simulink subsystem "moteur_bras_brushless"  (R2024a)
settings: Solver=VariableStepAuto  StartTime=0.0  StopTime=10.0  RelTol=1e-3
undefined symbols (not defined in the file): C_ref, Jv, rpm__max, Vref
libraries: fl_lib x22, fl_ps_legacy_lib x16, nesl_utility x15, sdl_lib x1, ee_lib x1
settings Model: Creator=vincp  LastModifiedBy=VincentPERRET

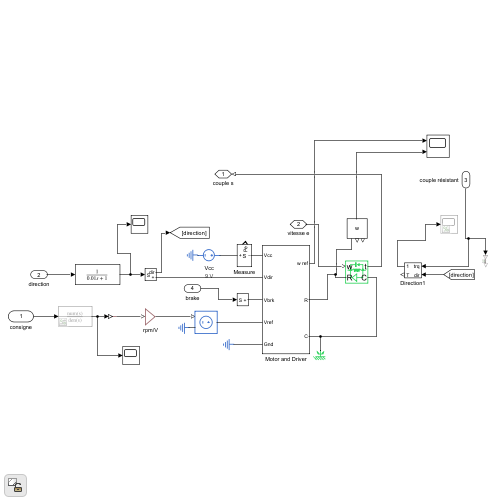
[thumbnail: Simulink's stored preview of the top-level diagram]
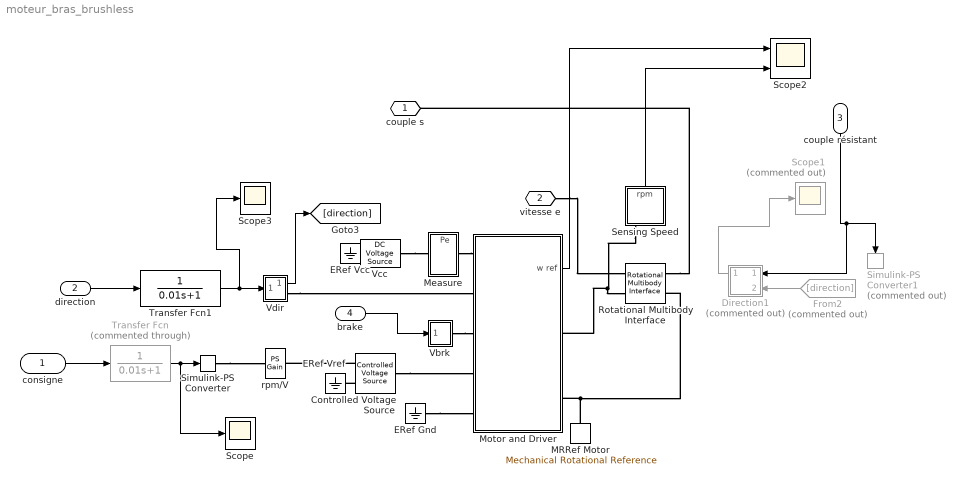
== system moteur_bras_brushless ==
  consigne : Inport
  direction : Inport  Port=2
  couple résistant : Inport  Port=3
  brake : Inport  Port=4
  Controlled Voltage Source : fl_lib/Electrical/Electrical Sources/Controlled Voltage Source
  Direction1 : Subsystem  Commented=on
  ERef Vcc : fl_lib/Electrical/Electrical Elements/Electrical Reference
  ERef Vref : fl_lib/Electrical/Electrical Elements/Electrical Reference
  ERef Gnd : fl_lib/Electrical/Electrical Elements/Electrical Reference
  From2 : From  Commented=on  GotoTag=direction
  MRRef Motor : fl_lib/Mechanical/Rotational Elements/Mechanical Rotational Reference
  Measure : Subsystem
      settings: PortSchema="{\"entries\":[{\"content\":{\"sides\":[{\"content\":{\"connectorIds\":[\"LConn1\"]},\"type\":\"ConnectorPlacement.EquallySpacedRectSide\",\"uuid\":\"8701fb7a-b552-4b0f-ba6a-9ffd5f92813c\"},{\"content\":{\"connectorIds\":[\"RConn1\"],\"side\":\"RIGHT\"},\"type\":\"ConnectorPlacement.EquallySpacedRectSide\",\"uuid\":\"c50126bd-8d71-4912-8eb9-bd6b1a4f4141\"},{\"content\":{\"connectorIds\":[\"Out1\"],\"side\":\"TOP\"},\"type\":\"ConnectorPlacement.EquallySpacedRectSide\",\"uuid\":\"9d2639c5-7e76-4bbd-8c8b-b1e420468010\"}]},\"type\":\"ConnectorPlacement.EquallySpacedConnector\",\"uuid\":\"8f301b36-1aea-45f7-af75-0d57371597bc\"}],\"packageUris\":[\"http://schema.mathworks.com/mf0/Connector/R2020b\"],\"version\":\"1.0\"}"
      mask Display: disp('S');
  Motor and Driver : Subsystem  Tag=PublishSubsystem  mask(Servomotor & Driver){Vcc=12, I0=44e-3, T_i=0.5e-3, eta=41, rpm_eta=40000, trq_eta=0.26e-3, trq_stall=0.44e-3, Kp=0.01, Ki=0.0001, Vref_max=5, rpm_max=rpm__max, J=Jv, rpm0=0}
      mask prompts: Vcc "Nominal voltage (V)"; I0 "No-load DC current to driver (A)"; T_i "Current loop time constant (s)"; eta "Efficiency (%)"; rpm_eta "Speed at which efficiency measured (rpm)"; trq_eta "Torque at which efficiency measured  (Nm)"; trq_stall "Stall torque (Nm)"; Kp "Proportional gain"; Ki "Integral gain"; Vref_max "Maximum reference voltage (V)"; rpm_max "Speed at maximum reference voltage (rpm)"; J "Rotor inerita (kg*m^2)"; rpm0 "Rotor initial speed (rpm)"
      mask help: Implements an abstracted model of a servomotor and driver configured for closed-loop speed control.
      mask DialogControl ParameterTabVar0 Prompt: Electrical
      mask DialogControl ParameterTabVar01 Prompt: Efficiency
      mask DialogControl ParameterTabVar012 Prompt: Mechanical
      mask DialogControl ParameterTabVar0123 Prompt: Controller
  Rotational Multibody Interface : fl_lib/Mechanical/Multibody Interfaces/Rotational Multibody Interface
  Scope : Scope
  Scope1 : Scope  Commented=on
  Scope2 : Scope  NumInputPorts=2
  Scope3 : Scope
  Sensing Speed : Subsystem
      mask Display: disp('w')
  Simulink-PS Converter : nesl_utility/Simulink-PS Converter  PhysicalDomain=network_engine_domain  SubClassName=ps_input  LeftPortType=input  RightPortType=output  PseudoPeriodic=off  Frequencies=[]  NoiseDistribution=none  NoiseParameters=[]  Unit=1  AffineConversion=off  FilteringAndDerivatives=zero  SimscapeFilterOrder=2  InputFilterTimeConstant=0.001  UdotUserProvided=0
  Simulink-PS Converter1 : nesl_utility/Simulink-PS Converter  Commented=on  PhysicalDomain=network_engine_domain  SubClassName=ps_input  LeftPortType=input  RightPortType=output  PseudoPeriodic=off  Frequencies=[]  NoiseDistribution=none  NoiseParameters=[]  Unit=N*m  AffineConversion=off  FilteringAndDerivatives=filter  SimscapeFilterOrder=2  InputFilterTimeConstant=0.001  UdotUserProvided=0
  Transfer Fcn : TransferFcn  Commented=through  Denominator=[0.01 1]
  Transfer Fcn1 : TransferFcn  Denominator=[0.01 1]
  Vbrk : Subsystem
      settings: CopyFcn=set_param(gcb,'LinkStatus','none')
  Vcc : fl_lib/Electrical/Electrical Sources/DC Voltage Source  v0=9 V
      settings: AttributesFormatString=%<v0> %<v0_unit>
  Vdir : Subsystem
      settings: CopyFcn=set_param(gcb,'LinkStatus','none')
  rpm/V : fl_ps_legacy_lib/Legacy Physical Signals/Functions/PS Gain  gain=Vref/rpm__max
  couple s : PMIOPort  Side=Left
  vitesse e : PMIOPort  Port=2  Side=Left
  wires:
  direction/1 -> Transfer Fcn1/1
  Transfer Fcn/1 -> Simulink-PS Converter/1, Scope/1
  Vdir/1(dir) -> [direction]
  From2/1 -> Direction1/2(dir)
  consigne/1 -> Transfer Fcn/1
  Direction1/1(Output) -> Scope1/1
  couple résistant/1 -> Direction1/1(trq), Simulink-PS Converter1/1
  Transfer Fcn1/1 -> Vdir/1(S), Scope3/1
  brake/1 -> Vbrk/1(S)
  Motor and Driver/1(w ref) -> Scope2/1
  Sensing Speed/1(rpm) -> Scope2/2
  connections:
  Sensing Speed/LConn1 -- Motor and Driver/RConn1 -- Rotational Multibody Interface/RConn2
  Rotational Multibody Interface/LConn2 -- MRRef Motor/LConn1 -- Motor and Driver/RConn2
  Controlled Voltage Source/RConn2 -- ERef Vref/LConn1
  Simulink-PS Converter/RConn1 -- rpm/V/LConn1
  Controlled Voltage Source/LConn1 -- Motor and Driver/LConn4
  ERef Vcc/LConn1 -- Vcc/RConn1
  Vcc/LConn1 -- Measure/LConn1
  ERef Gnd/LConn1 -- Motor and Driver/LConn5
  Measure/RConn1 -- Motor and Driver/LConn1
  Vdir/RConn1 -- Motor and Driver/LConn2
  Vbrk/RConn1 -- Motor and Driver/LConn3
  Controlled Voltage Source/RConn1 -- rpm/V/RConn1
  Rotational Multibody Interface/LConn1 -- couple s/RConn1
  vitesse e/RConn1 -- Rotational Multibody Interface/RConn1

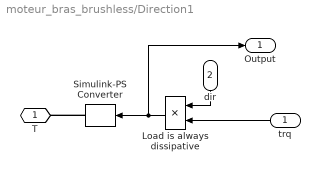
== system moteur_bras_brushless/Direction1 ==
  trq : Inport
  dir : Inport  Port=2
  Load is always dissipative : Product  InputSameDT=on  SaturateOnIntegerOverflow=on  OutDataTypeStr=Inherit: Same as first input
  Simulink-PS Converter : nesl_utility/Simulink-PS Converter  PhysicalDomain=network_engine_domain  SubClassName=ps_input  LeftPortType=input  RightPortType=output  PseudoPeriodic=off  Frequencies=[]  NoiseDistribution=none  NoiseParameters=[]  Unit=1  AffineConversion=off  FilteringAndDerivatives=zero  SimscapeFilterOrder=1  InputFilterTimeConstant=.001  UdotUserProvided=0
  T : PMIOPort  Side=Right
  Output : Outport
  wires:
  dir/1 -> Load is always dissipative/1
  trq/1 -> Load is always dissipative/2
  Load is always dissipative/1 -> Simulink-PS Converter/1, Output/1
  connections:
  Simulink-PS Converter/RConn1 -- T/RConn1

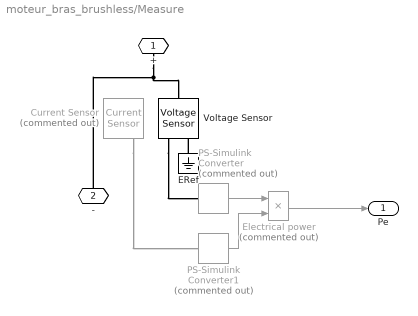
== system moteur_bras_brushless/Measure ==
  Current Sensor : fl_lib/Electrical/Electrical Sensors/Current Sensor  Commented=on
  ERef : fl_lib/Electrical/Electrical Elements/Electrical Reference
  Electrical power : Product  Commented=on  InputSameDT=on  SaturateOnIntegerOverflow=on  OutDataTypeStr=Inherit: Same as first input
  PS-Simulink Converter : nesl_utility/PS-Simulink Converter  Commented=on  PhysicalDomain=network_engine_domain  SubClassName=ps_output  LeftPortType=input  RightPortType=output  PseudoPeriodic=off  Frequencies=[]  VectorFormat=1-D array  Unit=V  AffineConversion=off
  PS-Simulink Converter1 : nesl_utility/PS-Simulink Converter  Commented=on  PhysicalDomain=network_engine_domain  SubClassName=ps_output  LeftPortType=input  RightPortType=output  PseudoPeriodic=off  Frequencies=[]  VectorFormat=1-D array  Unit=A  AffineConversion=off
  Voltage Sensor : fl_lib/Electrical/Electrical Sensors/Voltage Sensor
  + : PMIOPort  Side=Left
  - : PMIOPort  Port=2  Side=Right
  Pe : Outport
  wires:
  Electrical power/1 -> Pe/1
  PS-Simulink Converter1/1 -> Electrical power/2
  PS-Simulink Converter/1 -> Electrical power/1
  connections:
  Current Sensor/RConn1 -- PS-Simulink Converter1/LConn1
  ERef/LConn1 -- Voltage Sensor/RConn2
  Voltage Sensor/RConn1 -- PS-Simulink Converter/LConn1
  -/RConn1 -- +/RConn1 -- Voltage Sensor/LConn1

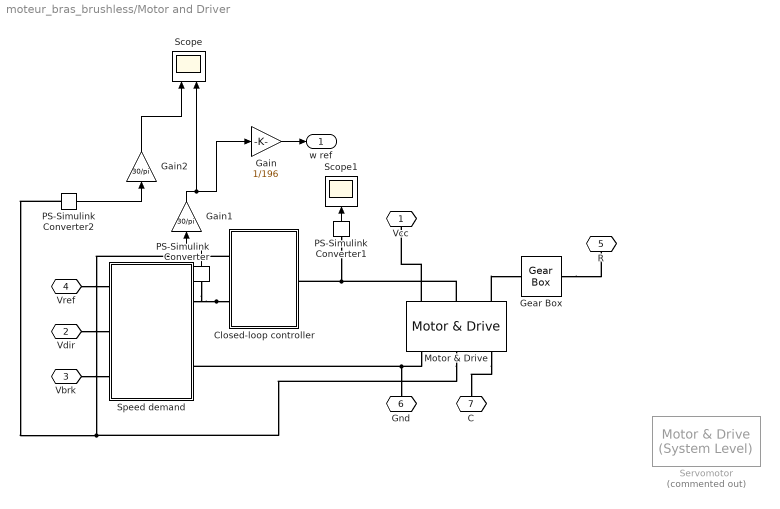
== system moteur_bras_brushless/Motor and Driver ==
  Closed-loop controller : Subsystem
  Gain : Gain  Gain=1/196
  Gain1 : Gain  Gain=30/pi
  Gain2 : Gain  Gain=30/pi
  Gear Box : fl_lib/Mechanical/Mechanisms/Gear Box  ratio=r_bras  t_in_specify=off  t_in_priority=None  t_in=0 N*m  t_in_nominal_specify=off  t_in_nominal_value=1  t_in_nominal_unit=N*m  t_out_specify=off  t_out_priority=None  t_out=0 N*m  t_out_nominal_specify=off  t_out_nominal_value=1  t_out_nominal_unit=N*m
  Motor & Drive : sdl_lib/Engines & Motors/Motor & Drive  torque_max=0.1 N*m  power_max=200 W  Tc=0.02 s  eff=100  w_eff=3750 rpm  T_eff=100 N*m  thermal_port=simscape.enum.thermaleffects.omit  thermal_mass=100 J/K  temperature_specify=off  temperature_priority=High  temperature=300 K  temperature_nominal_specify=off  temperature_nominal_value=1  temperature_nominal_unit=K
      settings: InternalSimscapePortConfiguration="{\"Bottom\":[],\"Left\":[{\"id\":\"Vp\",\"label\":\"+\",\"type\":\"foundation.electrical.electrical\"},{\"id\":\"Tr\",\"label\":\"Tr\",\"type\":\"input\"},{\"id\":\"R\",\"label\":\"R\",\"type\":\"foundation.mechanical.rotational.rotational\"}],\"Right\":[{\"id\":\"Vm\",\"label\":\"-\",\"type\":\"foundation.electrical.electrical\"},{\"id\":\"Omega\",\"label\":\"w\",\"type\":\"output\"},{\"id\":\"C\",\"label\":\"C\",\"type\":\"foundation.mechanical.rotational.rotational\"}],\"Top\":[]}"
  PS-Simulink Converter : nesl_utility/PS-Simulink Converter  PhysicalDomain=network_engine_domain  SubClassName=ps_output  LeftPortType=input  RightPortType=output  PseudoPeriodic=off  Frequencies=[]  VectorFormat=inherit  Unit=inherit  AffineConversion=off
  PS-Simulink Converter1 : nesl_utility/PS-Simulink Converter  PhysicalDomain=network_engine_domain  SubClassName=ps_output  LeftPortType=input  RightPortType=output  PseudoPeriodic=off  Frequencies=[]  VectorFormat=inherit  Unit=inherit  AffineConversion=off
  PS-Simulink Converter2 : nesl_utility/PS-Simulink Converter  PhysicalDomain=network_engine_domain  SubClassName=ps_output  LeftPortType=input  RightPortType=output  PseudoPeriodic=off  Frequencies=[]  VectorFormat=inherit  Unit=inherit  AffineConversion=off
  Scope : Scope  NumInputPorts=2
  Scope1 : Scope
  Servomotor : ee_lib/Electromechanical/Motor & Drive (System Level)  Commented=on  torque_speed_param=ee.enum.electromech.envelope.torque_power  overtorque_param=ee.enum.electromech.overtorque.no  T_t="[ C_ref C_ref C_ref  0 ] N*m"  T_t_intermittent=[.36, .32, .28, 0] N*m  T_t_2D=[.09, .09, .09; .08, .08, .08; .07, .07, .07; 0, 0, 0] N*m  T_t_intermittent_2D=[.36, .36, .36; .32, .32, .32; .28, .28, .28; 0, 0, 0] N*m  w_t="[  0 rpm__max 2*rpm__max 2.1*rpm__max ] rpm"  vdc_t=[6, 12, 24] V  torque_max=0.1 N*m  power_max=500 W  torque_max_intermittent=0.4 N*m  power_max_intermittent=120 W  time_overtorque=30 s  time_recover=60 s  Tc=T_i s  EnableSwitch=false  losses_param=1  eff=eta  w_eff=rpm_eta rpm  T_eff=trq_eta N*m  Piron=0 W  Pbase=Vcc*I0 W  w_eff_vec=[-8000 -4000 0 4000 8000] rpm  T_eff_vec=[0 0.03 0.06 0.09] N*m  v_eff_vec=[100, 250, 400] V  losses_mat=[1.49 1.67 2.21 3.10; 0.42 0.69 1.14 2.03; 0.06 0.24 0.78 1.68; 0.42 0.69 1.14 2.03; 1.49 1.67 2.21 3.10] W  efficiency_mat=[95 95 95 95; 95 95 95 95; 95 95 95 95; 95 95 95 95; 95 95 95 95]  losses_mat_3D=ones(5, 4, 3) W  efficiency_mat_3D=95 * ones(5, 4, 3)  Res=0 Ohm  enable_fault=simscape.enum.onoff.off  fault_condition=1  fault_threshold=0.5  J=Jv g*cm^2  lam=f N*m/(rad/s)  speed0=rpm0 rpm  faulted_specify=off  faulted_priority=None  faulted=0  faulted_nominal_specify=off  faulted_nominal_value=1  faulted_nominal_unit=1  isSwitchedOff_specify=off  isSwitchedOff_priority=None  isSwitchedOff=0  isSwitchedOff_nominal_specify=off  isSwitchedOff_nominal_value=1  isSwitchedOff_nominal_unit=1  torqueLimitContinuous_specify=off  torqueLimitContinuous_priority=None  torqueLimitContinuous=0 N*m  torqueLimitContinuous_nominal_specify=off  torqueLimitContinuous_nominal_value=1  torqueLimitContinuous_nominal_unit=N*m  alpha=3.93e-3 1/K  Tmeas=25 degC  Tmeas2=125 degC  losses_mat_T2=[1.49, 1.74, 2.49, 3.74; .42, .67, 1.42, 2.67; .06, .31, 1.06, 2.31; .42, .67, 1.42, 2.67; 1.49, 1.74, 2.49, 3.74] W  efficiency_mat_T2=[95, 95, 95, 95; 95, 95, 95, 95; 95, 95, 95, 95; 95, 95, 95, 95; 95, 95, 95, 95]  losses_mat_3D_T2=ones(5, 4, 3) W  efficiency_mat_3D_T2=95 * ones(5, 4, 3)  thermal_mass=100 J/K  initial_temperature=25 degC
  Speed demand : Subsystem
  Vcc : PMIOPort  Side=Left
  Vdir : PMIOPort  Port=2  Side=Left
  Vbrk : PMIOPort  Port=3  Side=Left
  Vref : PMIOPort  Port=4  Side=Left
  R : PMIOPort  Port=5  Side=Right
  Gnd : PMIOPort  Port=6  Side=Left
  C : PMIOPort  Port=7  Side=Right
  w ref : Outport
  wires:
  Gain2/1 -> Scope/1
  PS-Simulink Converter2/1 -> Gain2/1
  PS-Simulink Converter/1 -> Gain1/1
  Gain/1 -> w ref/1
  Gain1/1 -> Scope/2, Gain/1
  PS-Simulink Converter1/1 -> Scope1/1
  connections:
  Gear Box/RConn1 -- R/RConn1
  Closed-loop controller/LConn2 -- PS-Simulink Converter/LConn1 -- Speed demand/RConn1
  Motor & Drive/RConn2 -- Closed-loop controller/LConn1 -- PS-Simulink Converter2/LConn1
  Motor & Drive/LConn1 -- Vcc/RConn1
  Motor & Drive/LConn3 -- Gear Box/LConn1
  Vref/RConn1 -- Speed demand/LConn1
  Vdir/RConn1 -- Speed demand/LConn2
  Vbrk/RConn1 -- Speed demand/LConn3
  Motor & Drive/RConn1 -- Speed demand/RConn2 -- Gnd/RConn1
  Motor & Drive/RConn3 -- C/RConn1
  Motor & Drive/LConn2 -- PS-Simulink Converter1/LConn1 -- Closed-loop controller/RConn1

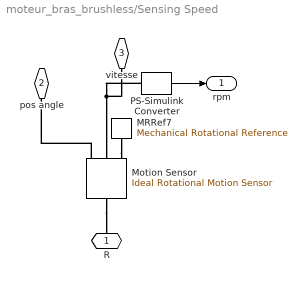
== system moteur_bras_brushless/Sensing Speed ==
  MRRef7 : fl_lib/Mechanical/Rotational Elements/Mechanical Rotational Reference
  Motion Sensor : fl_lib/Mechanical/Mechanical Sensors/Ideal Rotational Motion Sensor  reference=foundation.enum.MeasurementReference.difference  acceleration_port=false  velocity_port=true  position_port=true  wrap_angle=simscape.enum.onoff.off  offset=0 rad
  PS-Simulink Converter : nesl_utility/PS-Simulink Converter  PhysicalDomain=network_engine_domain  SubClassName=ps_output  LeftPortType=input  RightPortType=output  PseudoPeriodic=off  Frequencies=[]  VectorFormat=1-D array  Unit=rpm  AffineConversion=off
  R : PMIOPort  Side=Left
  pos angle : PMIOPort  Port=2  Side=Left
  vitesse : PMIOPort  Port=3  Side=Left
  rpm : Outport
  wires:
  PS-Simulink Converter/1 -> rpm/1
  connections:
  Motion Sensor/LConn1 -- R/RConn1
  MRRef7/LConn1 -- Motion Sensor/RConn1
  vitesse/RConn1 -- PS-Simulink Converter/LConn1 -- Motion Sensor/RConn2
  Motion Sensor/RConn3 -- pos angle/RConn1

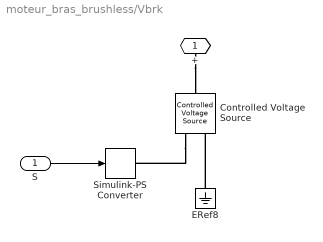
== system moteur_bras_brushless/Vbrk ==
  S : Inport
  Controlled Voltage Source : fl_lib/Electrical/Electrical Sources/Controlled Voltage Source
  ERef8 : fl_lib/Electrical/Electrical Elements/Electrical Reference
  Simulink-PS Converter : nesl_utility/Simulink-PS Converter  PhysicalDomain=network_engine_domain  SubClassName=ps_input  LeftPortType=input  RightPortType=output  PseudoPeriodic=off  Frequencies=[]  NoiseDistribution=none  NoiseParameters=[]  Unit=V  AffineConversion=off  FilteringAndDerivatives=zero  SimscapeFilterOrder=1  InputFilterTimeConstant=.001  UdotUserProvided=0
  + : PMIOPort  Side=Right
  wires:
  S/1 -> Simulink-PS Converter/1
  connections:
  Controlled Voltage Source/RConn1 -- Simulink-PS Converter/RConn1
  ERef8/LConn1 -- Controlled Voltage Source/RConn2
  +/RConn1 -- Controlled Voltage Source/LConn1

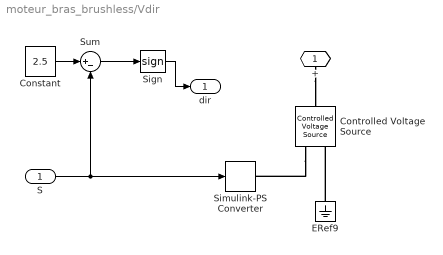
== system moteur_bras_brushless/Vdir ==
  S : Inport
  Constant : Constant  Value=2.5
  Controlled Voltage Source : fl_lib/Electrical/Electrical Sources/Controlled Voltage Source
  ERef9 : fl_lib/Electrical/Electrical Elements/Electrical Reference
  Sign : Signum
  Simulink-PS Converter : nesl_utility/Simulink-PS Converter  PhysicalDomain=network_engine_domain  SubClassName=ps_input  LeftPortType=input  RightPortType=output  PseudoPeriodic=off  Frequencies=[]  NoiseDistribution=none  NoiseParameters=[]  Unit=V  AffineConversion=off  FilteringAndDerivatives=zero  SimscapeFilterOrder=1  InputFilterTimeConstant=.001  UdotUserProvided=0
  Sum : Sum  Inputs=|+-  InputSameDT=on  SaturateOnIntegerOverflow=on  OutDataTypeStr=Inherit: Same as first input
  + : PMIOPort  Side=Right
  dir : Outport
  wires:
  Sign/1 -> dir/1
  Sum/1 -> Sign/1
  Constant/1 -> Sum/1
  S/1 -> Sum/2, Simulink-PS Converter/1
  connections:
  +/RConn1 -- Controlled Voltage Source/LConn1
  ERef9/LConn1 -- Controlled Voltage Source/RConn2
  Controlled Voltage Source/RConn1 -- Simulink-PS Converter/RConn1

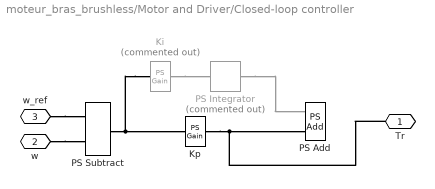
== system moteur_bras_brushless/Motor and Driver/Closed-loop controller ==
  Ki : fl_ps_legacy_lib/Legacy Physical Signals/Functions/PS Gain  Commented=on  gain=Ki
  Kp : fl_ps_legacy_lib/Legacy Physical Signals/Functions/PS Gain  gain=0.15
  PS Add : fl_ps_legacy_lib/Legacy Physical Signals/Functions/PS Add
      settings: InternalSimscapePortConfiguration="{\"Bottom\":[],\"Left\":[{\"id\":\"I1\",\"label\":\"\",\"type\":\"input\"},{\"id\":\"I2\",\"label\":\"\",\"type\":\"input\"}],\"Right\":[{\"id\":\"O\",\"label\":\"\",\"type\":\"output\"}],\"Top\":[]}"
  PS Integrator : fl_ps_legacy_lib/Legacy Physical Signals/Linear Operators/PS Integrator  Commented=on  x0=0
      settings: InternalSimscapePortConfiguration="{\"Bottom\":[],\"Left\":[{\"id\":\"I\",\"label\":\"\",\"type\":\"input\"}],\"Right\":[{\"id\":\"O\",\"label\":\"\",\"type\":\"output\"}],\"Top\":[]}"
  PS Subtract : fl_ps_legacy_lib/Legacy Physical Signals/Functions/PS Subtract
  Tr : PMIOPort  Side=Right
  w : PMIOPort  Port=2  Side=Left
  w_ref : PMIOPort  Port=3  Side=Left
  connections:
  Ki/LConn1 -- PS Subtract/RConn1 -- Kp/LConn1
  Ki/RConn1 -- PS Integrator/LConn1
  Tr/RConn1 -- Kp/RConn1 -- PS Add/LConn2
  PS Integrator/RConn1 -- PS Add/LConn1
  w_ref/RConn1 -- PS Subtract/LConn1
  w/RConn1 -- PS Subtract/LConn2

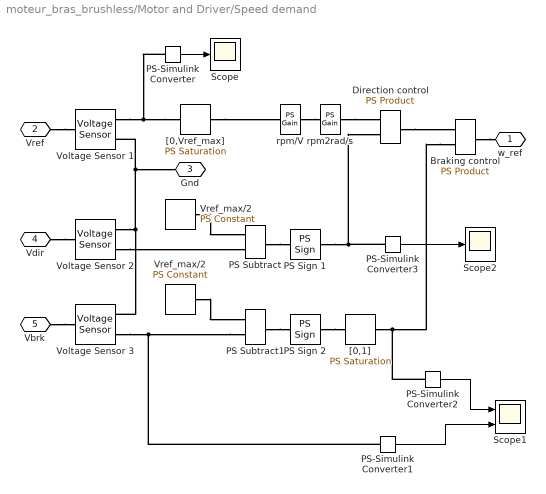
== system moteur_bras_brushless/Motor and Driver/Speed demand ==
  " Vref_max/2 " : fl_lib/Physical Signals/Sources/PS Constant  constant=Vref/2
  Braking control : fl_ps_legacy_lib/Legacy Physical Signals/Functions/PS Product
  Direction control : fl_ps_legacy_lib/Legacy Physical Signals/Functions/PS Product
  PS Sign 1 : fl_ps_legacy_lib/Legacy Physical Signals/Nonlinear Operators/PS Sign
      settings: InternalSimscapePortConfiguration="{\"Bottom\":[],\"Left\":[{\"id\":\"I\",\"label\":\"\",\"type\":\"input\"}],\"Right\":[{\"id\":\"O\",\"label\":\"\",\"type\":\"output\"}],\"Top\":[]}"
  PS Sign 2 : fl_ps_legacy_lib/Legacy Physical Signals/Nonlinear Operators/PS Sign
      settings: InternalSimscapePortConfiguration="{\"Bottom\":[],\"Left\":[{\"id\":\"I\",\"label\":\"\",\"type\":\"input\"}],\"Right\":[{\"id\":\"O\",\"label\":\"\",\"type\":\"output\"}],\"Top\":[]}"
  PS Subtract : fl_ps_legacy_lib/Legacy Physical Signals/Functions/PS Subtract
  PS Subtract1 : fl_ps_legacy_lib/Legacy Physical Signals/Functions/PS Subtract
  PS-Simulink Converter{,1..3} (4 alike) : nesl_utility/PS-Simulink Converter  PhysicalDomain=network_engine_domain  SubClassName=ps_output  LeftPortType=input  RightPortType=output  PseudoPeriodic=off  Frequencies=[]  VectorFormat=inherit  Unit=inherit  AffineConversion=off
  Scope : Scope
  Scope1 : Scope  NumInputPorts=2
  Scope2 : Scope
  Voltage Sensor 1 : fl_lib/Electrical/Electrical Sensors/Voltage Sensor
  Voltage Sensor 2 : fl_lib/Electrical/Electrical Sensors/Voltage Sensor
  Voltage Sensor 3 : fl_lib/Electrical/Electrical Sensors/Voltage Sensor
  Vref_max/2 : fl_lib/Physical Signals/Sources/PS Constant  constant=Vref/2
  "[0,1]" : fl_ps_legacy_lib/Legacy Physical Signals/Nonlinear Operators/PS Saturation  upper_limit=5  lower_limit=0
      settings: InternalSimscapePortConfiguration="{\"Bottom\":[],\"Left\":[{\"id\":\"I\",\"label\":\"\",\"type\":\"input\"}],\"Right\":[{\"id\":\"O\",\"label\":\"\",\"type\":\"output\"}],\"Top\":[]}"
  "[0,Vref_max]" : fl_ps_legacy_lib/Legacy Physical Signals/Nonlinear Operators/PS Saturation  upper_limit=Vref_max  lower_limit=0
      settings: InternalSimscapePortConfiguration="{\"Bottom\":[],\"Left\":[{\"id\":\"I\",\"label\":\"\",\"type\":\"input\"}],\"Right\":[{\"id\":\"O\",\"label\":\"\",\"type\":\"output\"}],\"Top\":[]}"
  rpm/V : fl_ps_legacy_lib/Legacy Physical Signals/Functions/PS Gain  gain=rpm__max/Vref
  rpm2rad/s : fl_ps_legacy_lib/Legacy Physical Signals/Functions/PS Gain  gain=2*pi/60
  w_ref : PMIOPort  Side=Right
  Vref : PMIOPort  Port=2  Side=Left
  Gnd : PMIOPort  Port=3  Side=Right
  Vdir : PMIOPort  Port=4  Side=Left
  Vbrk : PMIOPort  Port=5  Side=Left
  wires:
  PS-Simulink Converter3/1 -> Scope2/1
  PS-Simulink Converter1/1 -> Scope1/2
  PS-Simulink Converter2/1 -> Scope1/1
  PS-Simulink Converter/1 -> Scope/1
  connections:
  "[0,Vref_max]"/LConn1 -- PS-Simulink Converter/LConn1 -- Voltage Sensor 1/RConn1
  "[0,Vref_max]"/RConn1 -- rpm/V/LConn1
  rpm/V/RConn1 -- rpm2rad/s/LConn1
  Vref/RConn1 -- Voltage Sensor 1/LConn1
  Voltage Sensor 1/RConn2 -- Voltage Sensor 2/RConn2 -- Voltage Sensor 3/RConn2 -- Gnd/RConn1
  Vdir/RConn1 -- Voltage Sensor 2/LConn1
  PS Subtract/RConn1 -- PS Sign 1/LConn1
  rpm2rad/s/RConn1 -- Direction control/LConn1
  PS-Simulink Converter3/LConn1 -- PS Sign 1/RConn1 -- Direction control/LConn2
  Voltage Sensor 2/RConn1 -- PS Subtract/LConn2
  Vref_max/2/RConn1 -- PS Subtract/LConn1
  Vbrk/RConn1 -- Voltage Sensor 3/LConn1
  PS Subtract1/LConn2 -- PS-Simulink Converter1/LConn1 -- Voltage Sensor 3/RConn1
  " Vref_max/2 "/RConn1 -- PS Subtract1/LConn1
  PS Subtract1/RConn1 -- PS Sign 2/LConn1
  PS Sign 2/RConn1 -- "[0,1]"/LConn1
  Direction control/RConn1 -- Braking control/LConn1
  Braking control/RConn1 -- w_ref/RConn1
  Braking control/LConn2 -- PS-Simulink Converter2/LConn1 -- "[0,1]"/RConn1
